simulink model "LAB5"  (R2022b)
settings: Solver=VariableStepAuto  StartTime=0.0  StopTime=300  RelTol=1e-3
settings Model: PacingRate=11  Creator=zein  LastModifiedBy=zein

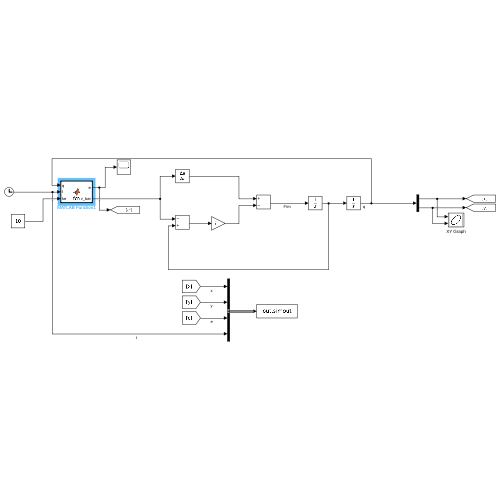
[thumbnail: Simulink's stored preview of the top-level diagram]
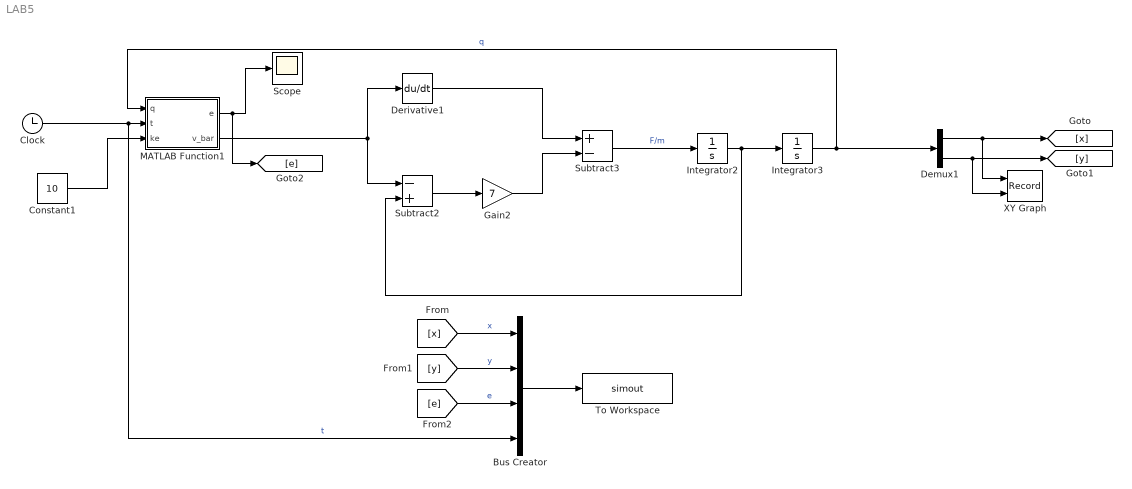
== system LAB5 ==
  Bus Creator : BusCreator  Inputs=4
  Clock : Clock
  Constant1 : Constant  Value=10
  Demux1 : Demux  Outputs=2
  Derivative1 : Derivative  CoefficientInTFapproximation=10
  Gain2 : Gain  Gain=7
  Integrator2 : Integrator
  Integrator3 : Integrator  InitialCondition=[-10;-4]
  MATLAB Function1 : MATLAB Function  TreatAsAtomicUnit=on
  Scope : Scope
  Subtract2 : Sum  Inputs=-+
  Subtract3 : Sum  Inputs=+-
  To Workspace : ToWorkspace  VariableName=simout  SaveFormat=Timeseries  SampleTime=-1
  XY Graph : Record  FileSettingsInternal="{\"entries\":[{\"content\":{\"excelSettings\":{\"content\":{},\"type\":\"Streamout.ExcelSettings\"}},\"type\":\"Streamout.FileSettingStorage\",\"uuid\":\"0ca1af2c-9ce1-40c9-a08a-d62fa3706bdb\"}],\"packageUris\":[\"http://schema.mathworks.com/mf0/streamout_blocks/R2020a\"],\"version\":\"1.0\"}"  Layout=[1 1]  SignalsInternal="{\"entries\":[{\"content\":{\"signals\":[{\"content\":{\"blockPath\":[\"LAB5/XY Graph\"],\"channel\":[],\"dimensions\":[1,1],\"domain\":\"LAB5/XY Graph\",\"lineColor\":\"#a2142f\",\"plots\":[1],\"port\":1,\"sid\":[\"\"],\"signalID\":19,\"signalName\":\"Demux1:1\"},\"type\":\"RecordBlkView.Signal\",\"uuid\":\"7c19cbd7-0587-451a-8c96-17d83656151c\"},{\"content\":{\"blockPath\":[\"LAB5/XY Graph\"],\"channel\":[],\"dimensions\":[1,1],\"domain\":\"LAB5/XY Graph\",\"lineColor\":\"#139fff\",\"plots\":[1],\"port\":2,\"sid\":[\"\"],\"signalID\":23,\"signalName\":\"Demux1:2\"},\"type\":\"RecordBlkView.Signal\",\"uuid\":\"d0812661-9dcd-410e-bf80-16d107bd6473\"}]},\"type\":\"RecordBlkView.InputSignals\",\"uuid\":\"b034e8f4-0afa-4b28-b8fd-25eaca2e2bd1\"}],\"packageUris\":[\"http://schema.mathworks.com/mf0/streamout_blocks/R2020a\"],\"version\":\"1.0\"}"  VisualizationBindings="{\"xyplotplugin\":{\"info\":[{\"series\":[{\"bindingParametersList\":[{\"parameter\":\"X-Axis\",\"signalID\":19,\"signalName\":\"Demux1:1\"},{\"parameter\":\"Y-Axis\",\"signalID\":23,\"signalName\":\"Demux1:2\"}],\"seriesID\":15178}],\"subplotID\":1}]}}"  CompatibilityTag=XY
  wires:
  Subtract2/1 -> Gain2/1
  Derivative1/1 -> Subtract3/1
  Gain2/1 -> Subtract3/2
  Subtract3/1 -> Integrator2/1  "F/m"
  Integrator2/1 -> Subtract2/2, Integrator3/1
  Constant1/1 -> MATLAB Function1/3(ke)
  Integrator3/1 -> MATLAB Function1/1(q), Demux1/1  "q"
  Demux1/2 -> XY Graph/2, [y]
  Demux1/1 -> XY Graph/1, [x]
  Clock/1 -> Bus Creator/4, MATLAB Function1/2(t)  "t"
  MATLAB Function1/2(v_bar) -> Derivative1/1, Subtract2/1
  MATLAB Function1/1(e) -> [e], Scope/1
  [x] -> Bus Creator/1  "x"
  [y] -> Bus Creator/2  "y"
  [e] -> Bus Creator/3  "e"
  Bus Creator/1 -> To Workspace/1

== matlab function LAB5/MATLAB Function1 ==
  data: e output; q input; t input; v_bar output; ke input
function [e, v_bar] = fcn(q, t, ke)

x = q(1);
y = q(2);

s_star = 2;
s = 2;


if(t<60*s_star/s)
    u_s = [(sqrt(2.0).*(x-y+2.0).*(-1.0./2.0))./(x.*1.4e+1+y.*1.0e+1+x.^2+y.^2+7.4e+1);
           (sqrt(2.0).*(x+y+1.2e+1).*(-1.0./2.0))./(x.*1.4e+1+y.*1.0e+1+x.^2+y.^2+7.4e+1)];

    u_e = [-ke.*(x.*2.0+1.4e+1).*((x+7.0).^2+(y+5.0).^2-2.5e+1./4.0);
           -ke.*(y.*2.0+1.0e+1).*((x+7.0).^2+(y+5.0).^2-2.5e+1./4.0)];

    e = (x+7)^2 + (y+5)^2 - 6.25;
elseif (t<80*s_star/s)
    u_s = [sqrt(2.0)./2.0+sqrt(6.0)./2.0;
          sqrt(2.0).*(-1.0./2.0)+sqrt(6.0)./2.0];

    u_e = [(sqrt(3.0).*ke.*(y./2.0-(sqrt(3.0).*x)./2.0+7.0./5.0))./2.0;
           ke.*(y./2.0-(sqrt(3.0).*x)./2.0+7.0./5.0).*(-1.0./2.0)];

    e = -sin(pi/3) * x + cos(pi/3) * y + 1.4;
else
    u_s = [(sqrt(2.0).*(x-y).*(-1.0./2.0))./(x.*-2.0e+1-y.*2.0e+1+x.^2+y.^2+2.0e+2);
           (sqrt(2.0).*(x+y-2.0e+1).*(-1.0./2.0))./(x.*-2.0e+1-y.*2.0e+1+x.^2+y.^2+2.0e+2)];

    u_e = [-ke.*(x.*2.0-2.0e+1).*((x-1.0e+1).^2+(y-1.0e+1).^2-3.6e+1);
           -ke.*(y.*2.0-2.0e+1).*((x-1.0e+1).^2+(y-1.0e+1).^2-3.6e+1)];

    e = (x-10)^2 + (y-10)^2 - 36 ;
end


v_bar = (s/s_star) * u_s + u_e;
